simulink subsystem "Orbit_Calculations"  (R2024b)
settings: Solver=VariableStepAuto  StartTime=0.0  StopTime=10.0  RelTol=1e-3
model mask{mu=0}
settings Model: Creator=cpero  LastModifiedBy=cpero

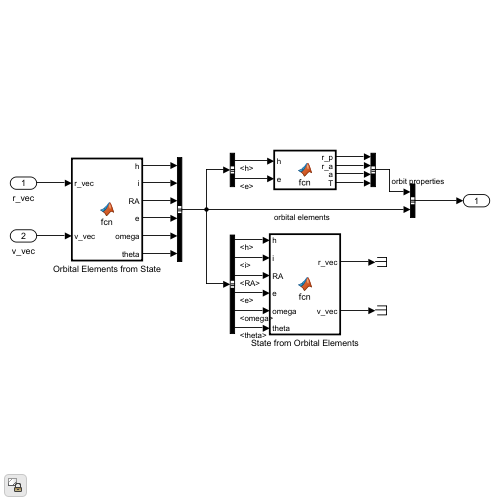
[thumbnail: Simulink's stored preview of the top-level diagram]
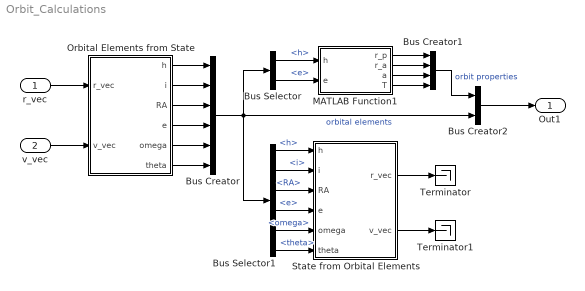
== system Orbit_Calculations ==
  r_vec : Inport
  v_vec : Inport  Port=2
  Bus Creator : BusCreator  Inputs=6
  Bus Creator1 : BusCreator  Inputs=4
  Bus Creator2 : BusCreator  Inputs=2
  Bus Selector : BusSelector  OutputSignals=h,e
  Bus Selector1 : BusSelector  OutputSignals=h,i,RA,e,omega,theta
  MATLAB Function1 : MATLAB Function  TreatAsAtomicUnit=on
  Orbital Elements from State : MATLAB Function  TreatAsAtomicUnit=on
  State from Orbital Elements : MATLAB Function  TreatAsAtomicUnit=on
  Terminator : Terminator
  Terminator1 : Terminator
  Out1 : Outport
  wires:
  Orbital Elements from State/4(e) -> Bus Creator/4
  Orbital Elements from State/6(theta) -> Bus Creator/6
  Bus Selector1/3 -> State from Orbital Elements/3(RA)  "<RA>"
  Orbital Elements from State/1(h) -> Bus Creator/1
  Orbital Elements from State/5(omega) -> Bus Creator/5
  Bus Creator/1 -> Bus Selector/1, Bus Creator2/2, Bus Selector1/1  "orbital elements"
  Bus Selector/2 -> MATLAB Function1/2(e)  "<e>"
  State from Orbital Elements/1(r_vec) -> Terminator/1
  Bus Selector/1 -> MATLAB Function1/1(h)  "<h>"
  Orbital Elements from State/3(RA) -> Bus Creator/3
  Bus Selector1/4 -> State from Orbital Elements/4(e)  "<e>"
  Bus Creator1/1 -> Bus Creator2/1  "orbit properties"
  MATLAB Function1/3(a) -> Bus Creator1/3
  Bus Selector1/5 -> State from Orbital Elements/5(omega)  "<omega>"
  v_vec/1 -> Orbital Elements from State/2(v_vec)
  Orbital Elements from State/2(i) -> Bus Creator/2
  Bus Selector1/6 -> State from Orbital Elements/6(theta)  "<theta>"
  Bus Creator2/1 -> Out1/1
  Bus Selector1/2 -> State from Orbital Elements/2(i)  "<i>"
  Bus Selector1/1 -> State from Orbital Elements/1(h)  "<h>"
  State from Orbital Elements/2(v_vec) -> Terminator1/1
  MATLAB Function1/2(r_a) -> Bus Creator1/2
  MATLAB Function1/1(r_p) -> Bus Creator1/1
  MATLAB Function1/4(T) -> Bus Creator1/4
  r_vec/1 -> Orbital Elements from State/1(r_vec)

== matlab function Orbit_Calculations/MATLAB Function1 ==
  data: h input; e input; r_p output; mu parameter; r_a output; a output; T output
function [r_p,r_a,a,T] = fcn(h, e, mu)

r_p = (h^2/mu)/(1+e);

if e < 1
    r_a = (h^2/mu)/(1-e);
    a = 0.5*(r_p + r_a);
    T = 2*pi*a^(3/2)/sqrt(mu);
else
    r_a = Inf;
    a = Inf;
    T = Inf;
end

== matlab function Orbit_Calculations/Orbital Elements from State ==
  data: r_vec input; h output; v_vec input; mu parameter; i output; RA output; e output; omega output; theta output
function [h,i,RA,e,omega,theta] = fcn(r_vec, v_vec, mu)

r = norm(r_vec);
v = norm(v_vec);
v_r = dot(r_vec, v_vec)/r;
h_vec = cross(r_vec,v_vec);
h = norm(h_vec);
i = acos(max(-1, min(h_vec(3)/h, 1)));
N_vec = cross([0;0;1],h_vec);
N = norm(N_vec);
RA = acos(N_vec(1)/N);
if N_vec(2) < 0
    RA = 2*pi - RA;
end
e_vec = (1/mu)*((v^2-(mu/r))*r_vec - r*v_r*v_vec);
e = norm(e_vec);
omega = acos(dot(N_vec,e_vec)/(N*e));
if e_vec(3) < 0
    omega = 2*pi - omega;
end
theta = acos(max(-1, min(dot(e_vec,r_vec)/(e*r), 1)));
if v_r < 0
    theta = 2*pi - theta;
end

== matlab function Orbit_Calculations/State from Orbital Elements ==
  data: h input; r_vec output; i input; RA input; e input; omega input; theta input; v_vec output; mu parameter
function [r_vec, v_vec] = fcn(h, i, RA, e, omega, theta, mu)

r_vec_peri = (h^2/mu)/(1+e*cos(theta))*[cos(theta);sin(theta);0];
v_vec_peri = (mu/h)*[-sin(theta); e+cos(theta); 0];
Q1 = [cos(omega), sin(omega), 0;
      -sin(omega), cos(omega), 0;
      0, 0, 1];
Q2 = [1, 0, 0;
      0, cos(i), sin(i);
      0, -sin(i), cos(i)];
Q3 = [cos(RA), sin(RA), 0;
      -sin(RA), cos(RA), 0;
      0, 0, 1];
peri2geo = (Q1*Q2*Q3)';
r_vec = peri2geo*r_vec_peri;
v_vec = peri2geo*v_vec_peri;
